simulink model "cungenz01"  (R2022a)
settings: Solver=VariableStepAuto  StartTime=0.0  StopTime=70  RelTol=1e-3
values from neighbouring files (symbols this model uses):
  cx = 0:0.1:120    [cungz_ref_01.m]
  cy = dy1/2.*(1+tanh(z1))-dy2/2.*(1+tanh(z2))    [cungz_ref_01.m]
libraries: Solver_SF x1, simulink x1
settings Model: Creator=wenju  LastModifiedBy=wenju

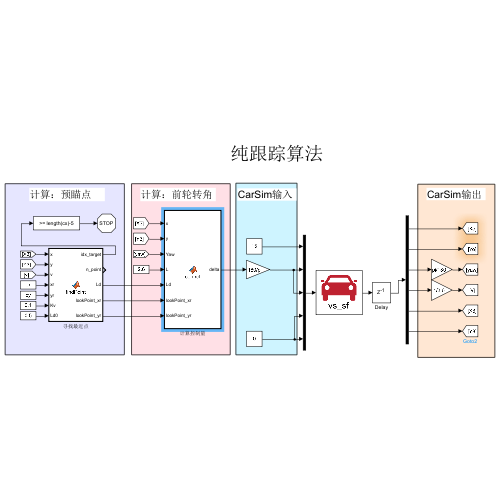
[thumbnail: Simulink's stored preview of the top-level diagram]
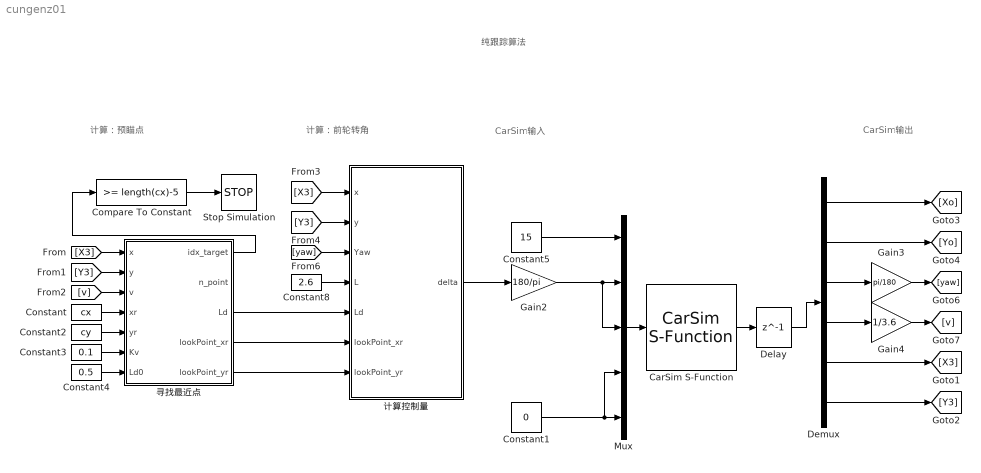
== system cungenz01 ==
  note: 计算：前轮转角
  note: CarSim输出
  note: 纯跟踪算法
  note: 计算：预瞄点
  note: CarSim输入
  CarSim S-Function : Solver_SF/CarSim S-Function  Priority=1  SIMFILE=simfile.sim  Run_RTs=off  vs_state_ind=Run  StopMode_ind=Vehicle Model
  Compare To Constant : simulink/Logic and Bit Operations/Compare To Constant  relop=>=  const=length(cx)-5  OutDataTypeStr=boolean
  Constant : Constant  Value=cx
  Constant1 : Constant  Value=0
  Constant2 : Constant  Value=cy
  Constant3 : Constant  Value=0.1
  Constant4 : Constant  Value=0.5
  Constant5 : Constant  Value=15
  Constant8 : Constant  Value=2.6
  Delay : Delay  DelayLength=1  InitialCondition=0  UseCircularBuffer=on
  Demux : Demux  Outputs=6
  Gain2 : Gain  Gain=180/pi
  Gain3 : Gain  Gain=pi/180
  Gain4 : Gain  Gain=1/3.6
  Mux : Mux  Inputs=5
  Stop Simulation : Stop
  寻找最近点 : MATLAB Function  TreatAsAtomicUnit=on
  计算控制量 : MATLAB Function  TreatAsAtomicUnit=on
  wires:
  CarSim S-Function/1 -> Delay/1
  Delay/1 -> Demux/1
  Mux/1 -> CarSim S-Function/1
  Constant1/1 -> Mux/4, Mux/5
  [v] -> 寻找最近点/3(v)
  Constant/1 -> 寻找最近点/4(xr)
  Constant2/1 -> 寻找最近点/5(yr)
  Constant3/1 -> 寻找最近点/6(Kv)
  Constant4/1 -> 寻找最近点/7(Ld0)
  [yaw] -> 计算控制量/3(Yaw)
  寻找最近点/1(idx_target) -> Compare To Constant/1
  寻找最近点/3(Ld) -> 计算控制量/5(Ld)
  寻找最近点/4(lookPoint_xr) -> 计算控制量/6(lookPoint_xr)
  寻找最近点/5(lookPoint_yr) -> 计算控制量/7(lookPoint_yr)
  计算控制量/1(delta) -> Gain2/1
  Constant8/1 -> 计算控制量/4(L)
  Gain2/1 -> Mux/3, Mux/2
  Compare To Constant/1 -> Stop Simulation/1
  Demux/3 -> Gain3/1
  Demux/4 -> Gain4/1
  Gain3/1 -> [yaw]
  Gain4/1 -> [v]
  Constant5/1 -> Mux/1
  Demux/5 -> [X3]
  Demux/6 -> [Y3]
  Demux/1 -> [Xo]
  Demux/2 -> [Yo]
  [X3] -> 寻找最近点/1(x)
  [Y3] -> 寻找最近点/2(y)
  [X3] -> 计算控制量/1(x)
  [Y3] -> 计算控制量/2(y)

== matlab function cungenz01/计算控制量 ==
  data: x input; y input; Yaw input; delta output; L input; Ld input; lookPoint_xr input; lookPoint_yr input
%% 获得控制量：前轮转向
function delta  = control(x,y,Yaw,L,Ld,lookPoint_xr,lookPoint_yr)
% 公式里的阿发角
alpha = atan2(lookPoint_yr - y,lookPoint_xr - x)  - Yaw;

% 前轮转角
delta = atan2(2*L*sin(alpha), Ld);
% 对前轮转角进行限制
if delta < -pi/3
   delta =  -pi/3;
end
if delta > pi/3
   delta = pi/3;
end

end

== matlab function cungenz01/寻找最近点 ==
  data: idx_target output; n_point output; Ld output; x input; y input; lookPoint_xr output; v input; xr input; yr input; Kv input; Ld0 input; lookPoint_yr output
%% 首先在参考轨迹上搜索离当前车辆位置最近的点
function  [idx_target,n_point,Ld,lookPoint_xr,lookPoint_yr] = findPoint(x,y, v,xr,yr, Kv, Ld0)

% 找到距离当前位置最近的一个参考轨迹点的序号
n=length(xr);
d_min=(x-xr(1))^2+(y-yr(1))^2;
min=0;
for i = 1:n
    d = (x-xr(i))^2+(y-yr(i))^2; 
    if d<d_min
        d_min=d;
        min=i;
    end
end

% 从该点开始向轨迹前方搜索，找到与预瞄距离最相近的一个轨迹点
L_steps = 0;           % 参考轨迹上几个相邻点的累计距离,从匹配点开始
Ld = Kv*v + Ld0;       % Ld0是预瞄距离的下限值；
    if min<=1
        
        min=1;
    end

while L_steps < Ld && min < n
    dx=xr(min+1) - xr(min);
    dy=yr(min+1) - yr(min);
    L_steps = L_steps + sqrt(dx^2+dy^2);
    min = min+1;
end
%找到与预瞄距离最相近的一个轨迹点索引号
idx_target = min;
n_point=n;
%从参考轨迹中给出目标点
lookPoint_xr = xr(idx_target);
lookPoint_yr = yr(idx_target);

end
